simulink model "exp8_3"  (R2023a)
settings: Solver=VariableStepAuto  StartTime=0.0  StopTime=10.0  RelTol=1e-3
libraries: simulink x2
settings Model: Creator=Lenovo  LastModifiedBy=zt

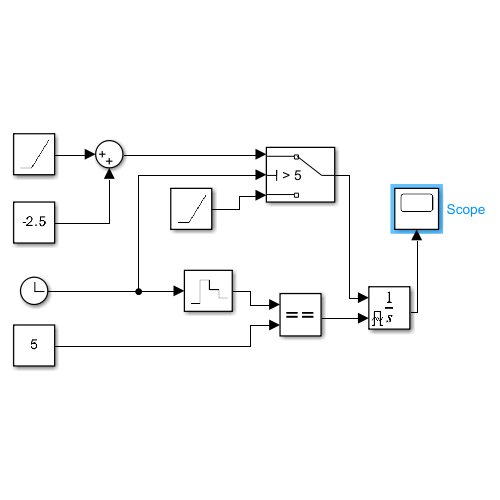
[thumbnail: Simulink's stored preview of the top-level diagram]
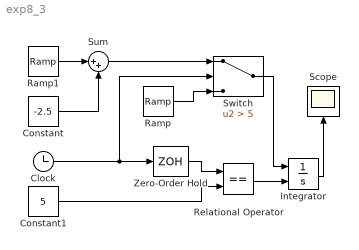
== system exp8_3 ==
  Clock : Clock
  Constant : Constant  Value=-2.5
  Constant1 : Constant  Value=5
  Integrator : Integrator  ExternalReset=either
  Ramp : simulink/Sources/Ramp  slope=0.5  start=0  InitialOutput=0
  Ramp1 : simulink/Sources/Ramp  slope=0.5  start=5  InitialOutput=0
  Relational Operator : RelationalOperator  Operator===  OutDataTypeStr=boolean  RndMeth=Simplest  InputSameDT=off
  Scope : Scope
  Sum : Sum  Inputs=|++
  Switch : Switch  Criteria=u2 > Threshold  Threshold=5  SaturateOnIntegerOverflow=off  InputSameDT=off
  Zero-Order Hold : ZeroOrderHold  SampleTime=1/1000
  wires:
  Ramp1/1 -> Sum/1
  Constant/1 -> Sum/2
  Clock/1 -> Switch/2, Zero-Order Hold/1
  Zero-Order Hold/1 -> Relational Operator/1
  Constant1/1 -> Relational Operator/2
  Relational Operator/1 -> Integrator/2
  Sum/1 -> Switch/1
  Ramp/1 -> Switch/3
  Switch/1 -> Integrator/1
  Integrator/1 -> Scope/1
